simulink model "lab1_model_betterPID"  (R2024b)
settings: Solver=ode45  StartTime=0.0  StopTime=sIn.time
undefined symbols (not defined in the file or in its folder): degs2rpm, drv, filt, gbox, mld, mot, PID, rads2rpm, rpm2degs, sens, sIn
libraries: simulink_extras x6, simulink x4
settings Model: Creator=bmm1  LastModifiedBy=pries
settings DataIOCC: ReturnWorkspaceOutputs=off
settings RTWCC: GPUComputeCapability=3.5

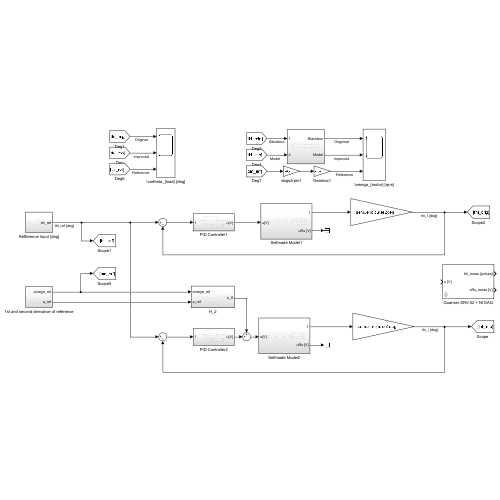
[thumbnail: Simulink's stored preview of the top-level diagram]
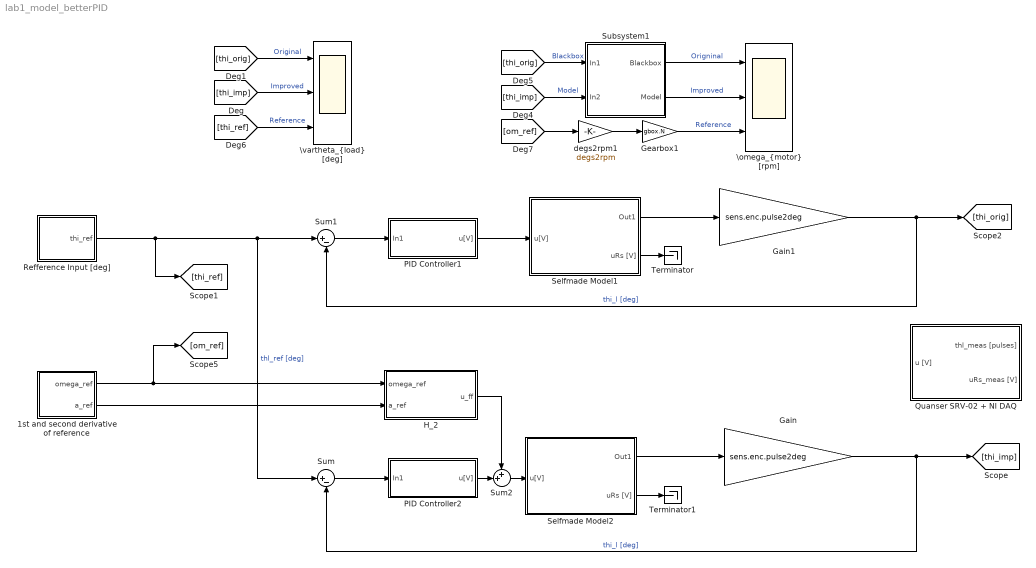
== system lab1_model_betterPID ==
  1st and second derivative of reference : Subsystem
  Gain : Gain  Gain=sens.enc.pulse2deg
  Gain1 : Gain  Gain=sens.enc.pulse2deg
  Gearbox1 : Gain  Gain=gbox.N
  H_2 : Subsystem
  PID Controller1 : Subsystem
  PID Controller2 : Subsystem
  Quanser SRV-02 + NI DAQ : Subsystem  mask(Quanser SRV-02 (with inertial load) + NI DAQ){Ts=0.001, fricType=Coulomb + viscous}
      mask prompts: Ts "NI DAQ Sample Time:"; fricType "Friction model"
      mask help: Quanser SRV-02 (with inertial load) + NI DAQ model.
      mask init:
      | %%  Sensors data
      | 
      | %   shunt resistor
      | sens.curr.Rs = 0.5;                         %   resistance [Ohm]   
      | sens.curr.uRs_std = 0.01;                   %   voltage noise standard dev [V]                           
      | sens.curr.uRs_var = sens.curr.uRs_std^2;	%   voltage noise variance [V^2]
      | 
      | %   Hewlett-Packard HEDS-5540#A06 optical encoder
      | sens.enc.ppr = 500*4;                       %   pulses per rotation
      | sens.enc.pulse2deg = 360/sens.enc.ppr;      %   [pulses] -> [deg]
      | sens.enc.pulse2rad = 2*pi/sens.enc.ppr;     %   [pulses] -> [rad]
      | sens.enc.deg2pulse = sens.enc.ppr/360;      %   [deg] -> [pulses]
      | sens.enc.rad2pulse = sens.enc.ppr/2/pi;     %   [rad] -> [pulses]
      | 
      | 
      | %%  Data acquisition board (daq) data
      | 
      | %   NI PCI-6221 DAC data
      | daq.dac.bits = 16;                                  %   resolution (bits)
      | daq.dac.fs   = 10;                                  %   full scale 
      | daq.dac.q    = 2*daq.dac.fs/(2^daq.dac.bits-1);     %	quantization
      | 
      | %   NI PCI-6221 ADC data
      | daq.adc.bits = 16;                                  %   resolution (bits)
      | daq.adc.fs   = 10;                                  %   full scale (as set in SLDRT Analog Input block)
      | daq.adc.q    = 2*daq.adc.fs/(2^daq.adc.bits-1);     %   quantization
      mask Help:
      | Riccardo Antonello (antonello@dei.unipd.it)
      | 
      | April 24, 2020
      | 
      | Dept. of Information Engineering, University of Padova
      mask TypeOptions fricType: Coulomb + viscous | Karnopp
  Refference Input [deg] : Subsystem
  Selfmade Model1 : Subsystem
  Selfmade Model2 : Subsystem
  Subsystem1 : Subsystem
  Sum : Sum  Inputs=|+-
  Sum1 : Sum  Inputs=|+-
  Sum2 : Sum  Inputs=++|
  Terminator : Terminator
  Terminator1 : Terminator
  "\\omega_{motor} [rpm]" : Scope  NumInputPorts=3
  "\\vartheta_{load} [deg]" : Scope  NumInputPorts=3
  degs2rpm1 : Gain  Gain=degs2rpm
  wires:
  Gain/1 -> Sum/2, [thi_imp]  "thi_l [deg]"
  Sum/1 -> PID Controller2/1(In1)
  Selfmade Model1/1(Out1) -> Gain1/1
  Gain1/1 -> Sum1/2, [thi_orig]  "thi_l [deg]"
  PID Controller1/1(u[V]) -> Selfmade Model1/1(u[V])
  Sum1/1 -> PID Controller1/1(In1)
  [thi_imp] -> "\\vartheta_{load} [deg]"/2  "Improved"
  Selfmade Model2/1(Out1) -> Gain/1
  [thi_orig] -> "\\vartheta_{load} [deg]"/1  "Original"
  Selfmade Model1/2(uRs [V]) -> Terminator/1
  Selfmade Model2/2(uRs [V]) -> Terminator1/1
  H_2/1(u_ff) -> Sum2/1
  PID Controller2/1(u[V]) -> Sum2/2
  Sum2/1 -> Selfmade Model2/1(u[V])
  [thi_imp] -> Subsystem1/2(In2)  "Model"
  [thi_orig] -> Subsystem1/1(In1)  "Blackbox"
  Subsystem1/1(Blackbox) -> "\\omega_{motor} [rpm]"/1  "Origninal"
  Subsystem1/2(Model) -> "\\omega_{motor} [rpm]"/2  "Improved"
  1st and second derivative of reference/1(omega_ref) -> [om_ref], H_2/1(omega_ref)
  1st and second derivative of reference/2(a_ref) -> H_2/2(a_ref)
  Refference Input [deg]/1(thi_ref) -> [thi_ref], Sum/1, Sum1/1  "thl_ref [deg]"
  [thi_ref] -> "\\vartheta_{load} [deg]"/3  "Reference"
  [om_ref] -> degs2rpm1/1
  Gearbox1/1 -> "\\omega_{motor} [rpm]"/3  "Reference"
  degs2rpm1/1 -> Gearbox1/1

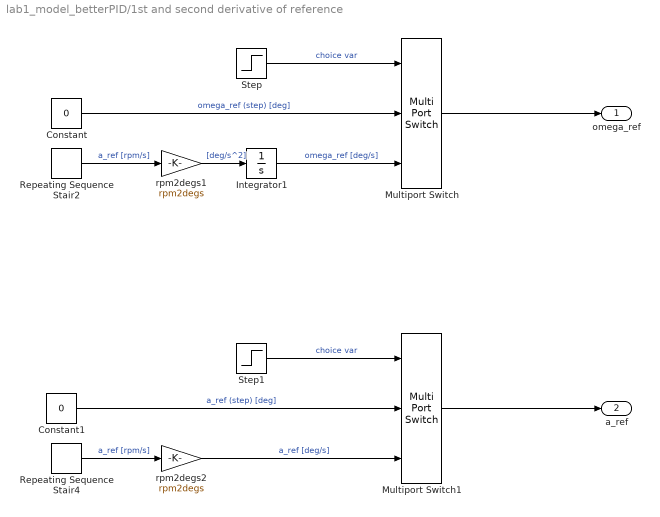
== system lab1_model_betterPID/1st and second derivative of reference ==
  Constant : Constant  Value=0
  Constant1 : Constant  Value=0
  Integrator1 : Integrator
  Multiport Switch : MultiPortSwitch  Inputs=2  SaturateOnIntegerOverflow=off  InputSameDT=off
  Multiport Switch1 : MultiPortSwitch  Inputs=2  SaturateOnIntegerOverflow=off  InputSameDT=off
  Repeating Sequence Stair2 : simulink/Sources/Repeating Sequence Stair  OutValues=feedforward.ref  tsamp=feedforward.time  OutMin=[]  OutMax=[]  OutDataTypeStr=double  OutputDataTypeScalingMode=double  OutDataType=fixdt(0,8)  ConRadixGroup=Best Precision: Vector-wise  OutScaling=2^-12
  Repeating Sequence Stair4 : simulink/Sources/Repeating Sequence Stair  OutValues=feedforward.ref  tsamp=feedforward.time  OutMin=[]  OutMax=[]  OutDataTypeStr=double  OutputDataTypeScalingMode=double  OutDataType=fixdt(0,8)  ConRadixGroup=Best Precision: Vector-wise  OutScaling=2^-12
  Step : Step  Time=0  After=sIn.program  SampleTime=0
  Step1 : Step  Time=0  After=sIn.program  SampleTime=0
  rpm2degs1 : Gain  Gain=rpm2degs
  rpm2degs2 : Gain  Gain=rpm2degs
  omega_ref : Outport
  a_ref : Outport  Port=2
  wires:
  Multiport Switch/1 -> omega_ref/1
  Multiport Switch1/1 -> a_ref/1
  Repeating Sequence Stair2/1 -> rpm2degs1/1  "a_ref [rpm/s]"
  Step/1 -> Multiport Switch/1  "choice var"
  Constant/1 -> Multiport Switch/2  "omega_ref (step) [deg]"
  rpm2degs1/1 -> Integrator1/1  "[deg/s^2]"
  Integrator1/1 -> Multiport Switch/3  "omega_ref [deg/s]"
  Repeating Sequence Stair4/1 -> rpm2degs2/1  "a_ref [rpm/s]"
  Step1/1 -> Multiport Switch1/1  "choice var"
  Constant1/1 -> Multiport Switch1/2  "a_ref (step) [deg]"
  rpm2degs2/1 -> Multiport Switch1/3  "a_ref [deg/s]"

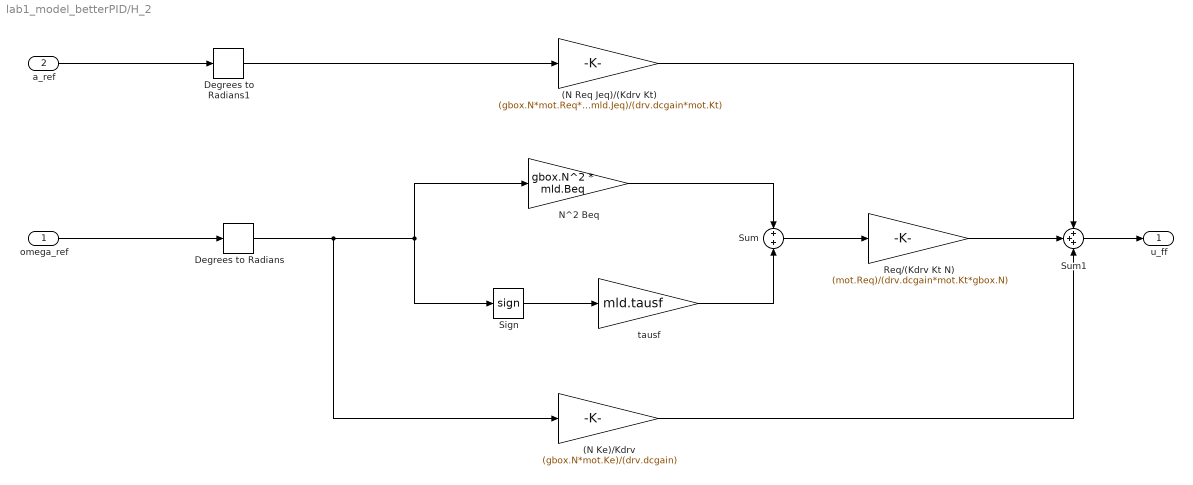
== system lab1_model_betterPID/H_2 ==
  omega_ref : Inport
  a_ref : Inport  Port=2
  (N Ke)/Kdrv : Gain  Gain=(gbox.N*mot.Ke)/(drv.dcgain)
  (N Req Jeq)/(Kdrv Kt) : Gain  Gain=(gbox.N*mot.Req*mld.Jeq)/(drv.dcgain*mot.Kt)
  Degrees to Radians : simulink_extras/Transformations/Degrees to Radians
  Degrees to Radians1 : simulink_extras/Transformations/Degrees to Radians
  N^2 Beq : Gain  Gain=gbox.N^2 * mld.Beq
  Req/(Kdrv Kt N) : Gain  Gain=(mot.Req)/(drv.dcgain*mot.Kt*gbox.N)
  Sign : Signum  ZeroCross=off
  Sum : Sum  Inputs=+|+
  Sum1 : Sum  Inputs=+++
  tausf : Gain  Gain=mld.tausf
  u_ff : Outport
  wires:
  tausf/1 -> Sum/2
  Sum/1 -> Req/(Kdrv Kt N)/1
  (N Ke)/Kdrv/1 -> Sum1/3
  Degrees to Radians/1 -> (N Ke)/Kdrv/1, Sign/1, N^2 Beq/1
  (N Req Jeq)/(Kdrv Kt)/1 -> Sum1/1
  N^2 Beq/1 -> Sum/1
  Req/(Kdrv Kt N)/1 -> Sum1/2
  Sign/1 -> tausf/1
  Degrees to Radians1/1 -> (N Req Jeq)/(Kdrv Kt)/1
  a_ref/1 -> Degrees to Radians1/1
  omega_ref/1 -> Degrees to Radians/1
  Sum1/1 -> u_ff/1

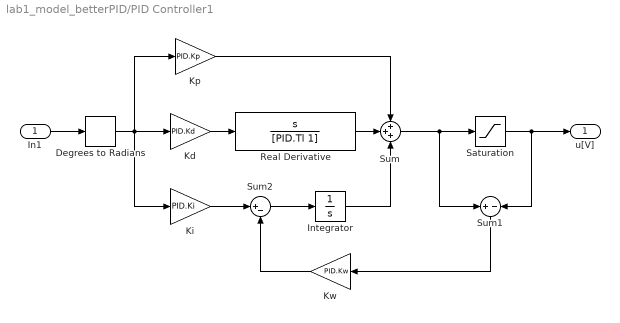
== system lab1_model_betterPID/PID Controller1 ==
  In1 : Inport
  Degrees to Radians : simulink_extras/Transformations/Degrees to Radians
  Integrator : Integrator
  Kd : Gain  Gain=PID.Kd
  Ki : Gain  Gain=PID.Ki
  Kp : Gain  Gain=PID.Kp
  Kw : Gain  Gain=PID.Kw
  Real Derivative : TransferFcn  Numerator=[1 0]  Denominator=[PID.Tl 1]
  Saturation : Saturate  UpperLimit=10  LowerLimit=-10
  Sum : Sum  Inputs=+++
  Sum1 : Sum  Inputs=+|-
  Sum2 : Sum  Inputs=|+-
  u[V] : Outport
  wires:
  In1/1 -> Degrees to Radians/1
  Sum/1 -> Sum1/1, Saturation/1
  Saturation/1 -> Sum1/2, u[V]/1
  Degrees to Radians/1 -> Ki/1, Kd/1, Kp/1
  Kd/1 -> Real Derivative/1
  Integrator/1 -> Sum/3
  Kp/1 -> Sum/1
  Real Derivative/1 -> Sum/2
  Ki/1 -> Sum2/1
  Sum2/1 -> Integrator/1
  Kw/1 -> Sum2/2
  Sum1/1 -> Kw/1

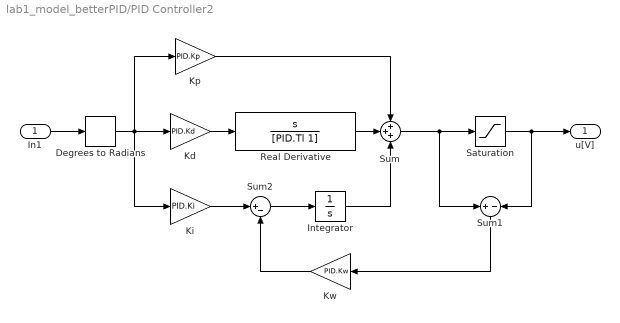
== system lab1_model_betterPID/PID Controller2 ==
  In1 : Inport
  Degrees to Radians : simulink_extras/Transformations/Degrees to Radians
  Integrator : Integrator
  Kd : Gain  Gain=PID.Kd
  Ki : Gain  Gain=PID.Ki
  Kp : Gain  Gain=PID.Kp
  Kw : Gain  Gain=PID.Kw
  Real Derivative : TransferFcn  Numerator=[1 0]  Denominator=[PID.Tl 1]
  Saturation : Saturate  UpperLimit=10  LowerLimit=-10
  Sum : Sum  Inputs=+++
  Sum1 : Sum  Inputs=+|-
  Sum2 : Sum  Inputs=|+-
  u[V] : Outport
  wires:
  In1/1 -> Degrees to Radians/1
  Sum/1 -> Sum1/1, Saturation/1
  Saturation/1 -> Sum1/2, u[V]/1
  Degrees to Radians/1 -> Ki/1, Kd/1, Kp/1
  Kd/1 -> Real Derivative/1
  Integrator/1 -> Sum/3
  Kp/1 -> Sum/1
  Real Derivative/1 -> Sum/2
  Ki/1 -> Sum2/1
  Sum2/1 -> Integrator/1
  Kw/1 -> Sum2/2
  Sum1/1 -> Kw/1

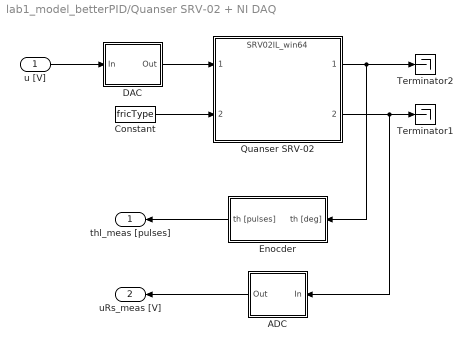
== system lab1_model_betterPID/Quanser SRV-02 + NI DAQ ==
  u [V] : Inport
  ADC : Subsystem
  Constant : Constant  Value=fricType
  DAC : Subsystem
  Enocder : Subsystem
  Quanser SRV-02 : ModelReference  ModelNameDialog=SRV02IL_win64.slxp  ModelReferenceVersion=1.44  CopyOfModelProtected=on
  Terminator1 : Terminator
  Terminator2 : Terminator
  thl_meas [pulses] : Outport
  uRs_meas [V] : Outport  Port=2
  wires:
  Enocder/1(th [pulses]) -> thl_meas [pulses]/1
  ADC/1(Out) -> uRs_meas [V]/1
  DAC/1(Out) -> Quanser SRV-02/1
  Quanser SRV-02/2 -> ADC/1(In), Terminator1/1
  u [V]/1 -> DAC/1(In)
  Quanser SRV-02/1 -> Enocder/1(th [deg]), Terminator2/1
  Constant/1 -> Quanser SRV-02/2

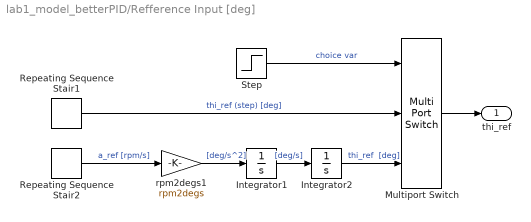
== system lab1_model_betterPID/Refference Input [deg] ==
  Integrator1 : Integrator
  Integrator2 : Integrator
  Multiport Switch : MultiPortSwitch  Inputs=2  SaturateOnIntegerOverflow=off  InputSameDT=off
  Repeating Sequence Stair1 : simulink/Sources/Repeating Sequence Stair  OutValues=windup.ref  tsamp=windup.time  OutMin=[]  OutMax=[]  OutDataTypeStr=double  OutputDataTypeScalingMode=double  OutDataType=fixdt(0,8)  ConRadixGroup=Best Precision: Vector-wise  OutScaling=2^-12
  Repeating Sequence Stair2 : simulink/Sources/Repeating Sequence Stair  OutValues=feedforward.ref  tsamp=feedforward.time  OutMin=[]  OutMax=[]  OutDataTypeStr=double  OutputDataTypeScalingMode=double  OutDataType=fixdt(0,8)  ConRadixGroup=Best Precision: Vector-wise  OutScaling=2^-12
  Step : Step  Time=0  After=sIn.program  SampleTime=0
  rpm2degs1 : Gain  Gain=rpm2degs
  thi_ref : Outport
  wires:
  Repeating Sequence Stair2/1 -> rpm2degs1/1  "a_ref [rpm/s]"
  rpm2degs1/1 -> Integrator1/1  "[deg/s^2]"
  Repeating Sequence Stair1/1 -> Multiport Switch/2  "thi_ref (step) [deg]"
  Integrator1/1 -> Integrator2/1  "[deg/s]"
  Step/1 -> Multiport Switch/1  "choice var"
  Integrator2/1 -> Multiport Switch/3  "thi_ref  [deg]"
  Multiport Switch/1 -> thi_ref/1

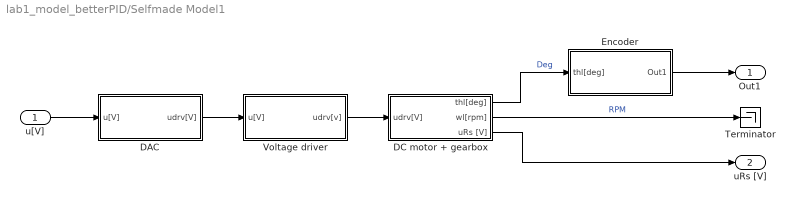
== system lab1_model_betterPID/Selfmade Model1 ==
  u[V] : Inport
  DAC : Subsystem
  DC motor + gearbox : Subsystem
  Encoder : Subsystem
  Terminator : Terminator
  Voltage driver : Subsystem
  Out1 : Outport
  uRs [V] : Outport  Port=2
  wires:
  DC motor + gearbox/3(uRs [V]) -> uRs [V]/1
  Encoder/1(Out1) -> Out1/1
  Voltage driver/1(udrv[v]) -> DC motor + gearbox/1(udrv[V])
  DAC/1(udrv[V]) -> Voltage driver/1(u[V])
  DC motor + gearbox/2(wl[rpm]) -> Terminator/1  "RPM"
  u[V]/1 -> DAC/1(u[V])
  DC motor + gearbox/1(thl[deg]) -> Encoder/1(thl[deg])  "Deg"

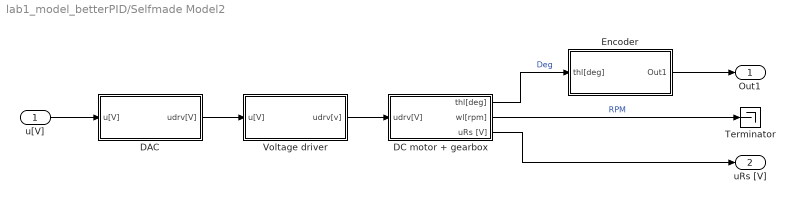
== system lab1_model_betterPID/Selfmade Model2 ==
  u[V] : Inport
  DAC : Subsystem
  DC motor + gearbox : Subsystem
  Encoder : Subsystem
  Terminator : Terminator
  Voltage driver : Subsystem
  Out1 : Outport
  uRs [V] : Outport  Port=2
  wires:
  DC motor + gearbox/1(thl[deg]) -> Encoder/1(thl[deg])  "Deg"
  u[V]/1 -> DAC/1(u[V])
  DC motor + gearbox/2(wl[rpm]) -> Terminator/1  "RPM"
  DAC/1(udrv[V]) -> Voltage driver/1(u[V])
  Voltage driver/1(udrv[v]) -> DC motor + gearbox/1(udrv[V])
  Encoder/1(Out1) -> Out1/1
  DC motor + gearbox/3(uRs [V]) -> uRs [V]/1

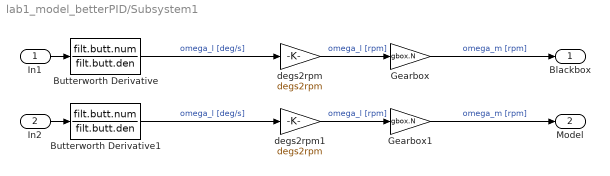
== system lab1_model_betterPID/Subsystem1 ==
  In1 : Inport
  In2 : Inport  Port=2
  Butterworth Derivative : TransferFcn  Numerator=filt.butt.num  Denominator=filt.butt.den
  Butterworth Derivative1 : TransferFcn  Numerator=filt.butt.num  Denominator=filt.butt.den
  Gearbox : Gain  Gain=gbox.N
  Gearbox1 : Gain  Gain=gbox.N
  degs2rpm : Gain  Gain=degs2rpm
  degs2rpm1 : Gain  Gain=degs2rpm
  Blackbox : Outport
  Model : Outport  Port=2
  wires:
  Gearbox/1 -> Blackbox/1  "omega_m [rpm]"
  In2/1 -> Butterworth Derivative1/1
  Butterworth Derivative1/1 -> degs2rpm1/1  "omega_l [deg/s]"
  In1/1 -> Butterworth Derivative/1
  degs2rpm1/1 -> Gearbox1/1  "omega_l [rpm]"
  degs2rpm/1 -> Gearbox/1  "omega_l [rpm]"
  Butterworth Derivative/1 -> degs2rpm/1  "omega_l [deg/s]"
  Gearbox1/1 -> Model/1  "omega_m [rpm]"

== system lab1_model_betterPID/Quanser SRV-02 + NI DAQ/ADC ==
  In : Inport
  Quantizer : Quantizer  QuantizationInterval=daq.adc.q
  Saturation : Saturate  UpperLimit=daq.adc.fs  LowerLimit=-daq.adc.fs
  Zero-Order Hold : ZeroOrderHold  SampleTime=Ts
  Out : Outport
  wires:
  Saturation/1 -> Out/1
  In/1 -> Zero-Order Hold/1
  Quantizer/1 -> Saturation/1
  Zero-Order Hold/1 -> Quantizer/1

== system lab1_model_betterPID/Quanser SRV-02 + NI DAQ/DAC ==
  In : Inport
  Quantizer : Quantizer  QuantizationInterval=daq.dac.q
  Saturation : Saturate  UpperLimit=daq.dac.fs  LowerLimit=-daq.dac.fs
  Zero-Order Hold : ZeroOrderHold  SampleTime=Ts
  Out : Outport
  wires:
  Quantizer/1 -> Saturation/1
  In/1 -> Zero-Order Hold/1
  Zero-Order Hold/1 -> Quantizer/1
  Saturation/1 -> Out/1

== system lab1_model_betterPID/Quanser SRV-02 + NI DAQ/Enocder ==
  th [deg] : Inport
  Quantizer : Quantizer  QuantizationInterval=sens.enc.pulse2deg
  Zero-Order Hold : ZeroOrderHold  SampleTime=Ts
  deg2pulse : Gain  Gain=sens.enc.deg2pulse
  th [pulses] : Outport
  wires:
  Quantizer/1 -> deg2pulse/1
  th [deg]/1 -> Zero-Order Hold/1
  Zero-Order Hold/1 -> Quantizer/1
  deg2pulse/1 -> th [pulses]/1

== system lab1_model_betterPID/Selfmade Model1/DAC ==
  u[V] : Inport
  Quantizer : Quantizer  QuantizationInterval=daq.dac.q
  Saturation : Saturate  UpperLimit=10  LowerLimit=-10
  Zero-Order Hold : ZeroOrderHold  SampleTime=1e-3
  udrv[V] : Outport
  wires:
  Saturation/1 -> udrv[V]/1
  Quantizer/1 -> Saturation/1
  u[V]/1 -> Zero-Order Hold/1
  Zero-Order Hold/1 -> Quantizer/1

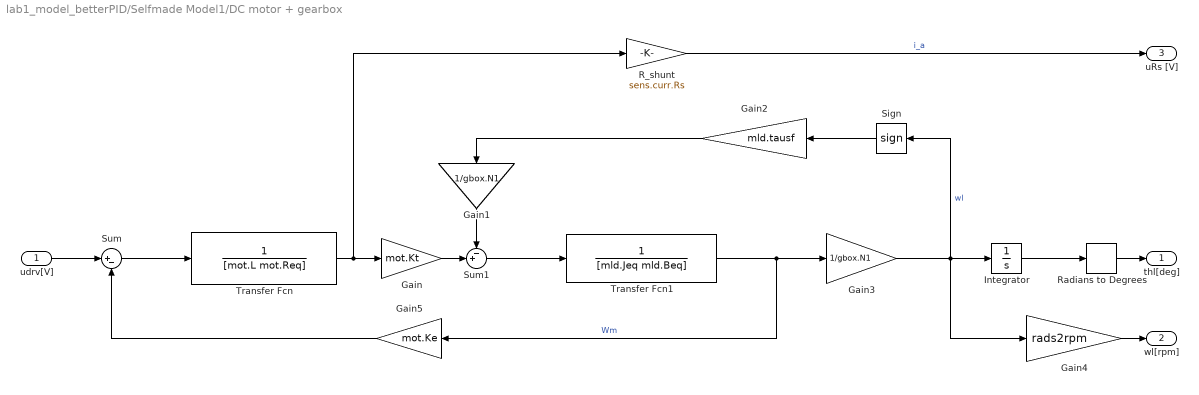
== system lab1_model_betterPID/Selfmade Model1/DC motor + gearbox ==
  udrv[V] : Inport
  Gain : Gain  Gain=mot.Kt
  Gain1 : Gain  Gain=1/gbox.N1
  Gain2 : Gain  Gain=mld.tausf
  Gain3 : Gain  Gain=1/gbox.N1
  Gain4 : Gain  Gain=rads2rpm
  Gain5 : Gain  Gain=mot.Ke
  Integrator : Integrator
  R_shunt : Gain  Gain=sens.curr.Rs
  Radians to Degrees : simulink_extras/Transformations/Radians to Degrees
  Sign : Signum  ZeroCross=off
  Sum : Sum  Inputs=|+-
  Sum1 : Sum  Inputs=-+|
  Transfer Fcn : TransferFcn  Denominator=[mot.L mot.Req]
  Transfer Fcn1 : TransferFcn  Denominator=[mld.Jeq mld.Beq]
  thl[deg] : Outport
  wl[rpm] : Outport  Port=2
  uRs [V] : Outport  Port=3
  wires:
  R_shunt/1 -> uRs [V]/1  "i_a"
  Gain5/1 -> Sum/2
  Gain/1 -> Sum1/2
  Sum1/1 -> Transfer Fcn1/1
  Gain4/1 -> wl[rpm]/1
  Radians to Degrees/1 -> thl[deg]/1
  Integrator/1 -> Radians to Degrees/1
  Gain3/1 -> Integrator/1, Sign/1, Gain4/1  "wl"
  Transfer Fcn1/1 -> Gain3/1, Gain5/1  "Wm"
  Sign/1 -> Gain2/1
  Gain2/1 -> Gain1/1
  Gain1/1 -> Sum1/1
  Transfer Fcn/1 -> Gain/1, R_shunt/1
  Sum/1 -> Transfer Fcn/1
  udrv[V]/1 -> Sum/1

== system lab1_model_betterPID/Selfmade Model1/Encoder ==
  thl[deg] : Inport
  Gain : Gain  Gain=1/sens.enc.pulse2deg
  Quantizer : Quantizer  QuantizationInterval=sens.enc.pulse2deg
  Zero-Order Hold : ZeroOrderHold  SampleTime=1e-3
  Out1 : Outport
  wires:
  Zero-Order Hold/1 -> Quantizer/1
  Quantizer/1 -> Gain/1
  Gain/1 -> Out1/1
  thl[deg]/1 -> Zero-Order Hold/1

== system lab1_model_betterPID/Selfmade Model1/Voltage driver ==
  u[V] : Inport
  Saturation : Saturate  UpperLimit=12  LowerLimit=-12
  Transfer Fcn : TransferFcn  Numerator=[drv.dcgain]  Denominator=[drv.Tc 1]
  udrv[v] : Outport
  wires:
  Saturation/1 -> udrv[v]/1
  Transfer Fcn/1 -> Saturation/1
  u[V]/1 -> Transfer Fcn/1

== system lab1_model_betterPID/Selfmade Model2/DAC ==
  u[V] : Inport
  Quantizer : Quantizer  QuantizationInterval=daq.dac.q
  Saturation : Saturate  UpperLimit=10  LowerLimit=-10
  Zero-Order Hold : ZeroOrderHold  SampleTime=1e-3
  udrv[V] : Outport
  wires:
  Zero-Order Hold/1 -> Quantizer/1
  u[V]/1 -> Zero-Order Hold/1
  Quantizer/1 -> Saturation/1
  Saturation/1 -> udrv[V]/1

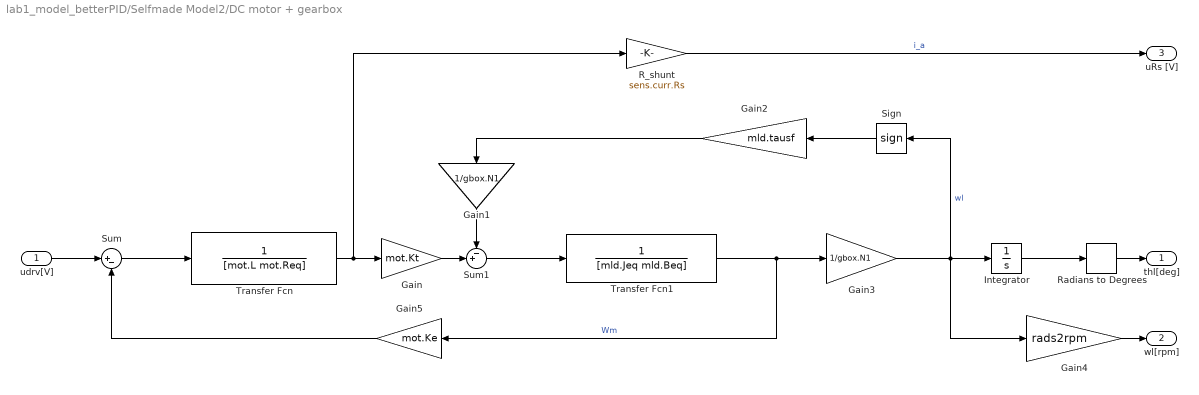
== system lab1_model_betterPID/Selfmade Model2/DC motor + gearbox ==
  udrv[V] : Inport
  Gain : Gain  Gain=mot.Kt
  Gain1 : Gain  Gain=1/gbox.N1
  Gain2 : Gain  Gain=mld.tausf
  Gain3 : Gain  Gain=1/gbox.N1
  Gain4 : Gain  Gain=rads2rpm
  Gain5 : Gain  Gain=mot.Ke
  Integrator : Integrator
  R_shunt : Gain  Gain=sens.curr.Rs
  Radians to Degrees : simulink_extras/Transformations/Radians to Degrees
  Sign : Signum  ZeroCross=off
  Sum : Sum  Inputs=|+-
  Sum1 : Sum  Inputs=-+|
  Transfer Fcn : TransferFcn  Denominator=[mot.L mot.Req]
  Transfer Fcn1 : TransferFcn  Denominator=[mld.Jeq mld.Beq]
  thl[deg] : Outport
  wl[rpm] : Outport  Port=2
  uRs [V] : Outport  Port=3
  wires:
  udrv[V]/1 -> Sum/1
  Sum/1 -> Transfer Fcn/1
  Transfer Fcn/1 -> R_shunt/1, Gain/1
  Gain1/1 -> Sum1/1
  Gain2/1 -> Gain1/1
  Sign/1 -> Gain2/1
  Transfer Fcn1/1 -> Gain5/1, Gain3/1  "Wm"
  Gain3/1 -> Gain4/1, Sign/1, Integrator/1  "wl"
  Integrator/1 -> Radians to Degrees/1
  Radians to Degrees/1 -> thl[deg]/1
  Gain4/1 -> wl[rpm]/1
  Sum1/1 -> Transfer Fcn1/1
  Gain/1 -> Sum1/2
  Gain5/1 -> Sum/2
  R_shunt/1 -> uRs [V]/1  "i_a"

== system lab1_model_betterPID/Selfmade Model2/Encoder ==
  thl[deg] : Inport
  Gain : Gain  Gain=1/sens.enc.pulse2deg
  Quantizer : Quantizer  QuantizationInterval=sens.enc.pulse2deg
  Zero-Order Hold : ZeroOrderHold  SampleTime=1e-3
  Out1 : Outport
  wires:
  thl[deg]/1 -> Zero-Order Hold/1
  Gain/1 -> Out1/1
  Quantizer/1 -> Gain/1
  Zero-Order Hold/1 -> Quantizer/1

== system lab1_model_betterPID/Selfmade Model2/Voltage driver ==
  u[V] : Inport
  Saturation : Saturate  UpperLimit=12  LowerLimit=-12
  Transfer Fcn : TransferFcn  Numerator=[drv.dcgain]  Denominator=[drv.Tc 1]
  udrv[v] : Outport
  wires:
  u[V]/1 -> Transfer Fcn/1
  Transfer Fcn/1 -> Saturation/1
  Saturation/1 -> udrv[v]/1
